simulink model "LabC_CompensatorOverRobot"  (R2020b)
settings: Solver=FixedStepDiscrete  StartTime=0.0  StopTime=inf  FixedStep=fSamplingPeriod  RelTol=1e-3  EnableMultiTasking=on
values from neighbouring files (symbols this model uses):
  acc_LSB_per_g = 16384    [GyroAccScaling.mat]
  acc_y_offset = 651.5    [OffsetData.mat]
  acc_z_offset = 170.75    [OffsetData.mat]
  Ad = Acl    [LabB_ObserverAndControllerOverSimulator_Discrete_Parameters.m]    (also in LabB_ObserverOverSimulator_Discrete_Parameters.m; LabC_6_4.m = Ad; LabC_6_5.m = Ad; LabC_6_6.m)
  Cd = [1,0,0,0 ; 0,0,1,0]    [LabB_ObserverAndControllerOverSimulator_Discrete_Parameters.m]    (also in LabB_ObserverOverSimulator_Discrete_Parameters.m; LabC_6_4.m; LabC_6_5.m; LabC_6_6.m = [1,0,0,0])
  fSamplingPeriod = 0.005    [LabB_ControllerOverSimulator_Discrete_Parameters.m]    (also in LabB_ControllerOverSimulator_Discrete_Parameters_conflict_copy_LAPTOP-FOGVCHE7_2020_11_15.m; LabB_ObserverAndControllerOverSimulator_Discrete_Parameters.m; LabC_6_3.m = 0.2; LabC_6_4.m = 0.067)
  fWheelRadius = 0.0216    [LoadRobotParameters.m]
  gyro_LSB_per_deg = 131    [GyroAccScaling.mat]
  gyro_x_offset = -193.125    [OffsetData.mat]
  iNumberOfEncoderSteps = 720    [LoadRobotParameters.m]
  Kd = place(Ad, Bd, Pd)    [LabB_ControllerOverSimulator_Discrete_Parameters.m]    (also in LabB_ControllerOverSimulator_Discrete_Parameters_conflict_copy_LAPTOP-FOGVCHE7_2020_11_15.m = c2d(K,fSamplingPeriod,'zoh'); LabB_ObserverAndControllerOverSimulator_Discrete_Parameters.m; LabC_6_6.m; LabC_CompensatorOverRobot_Parameters.m)
  Ld = (place(Ad',Cd',afPoles_full_d))'    [LabB_ObserverAndControllerOverSimulator_Discrete_Parameters.m]    (also in LabB_ObserverOverSimulator_Discrete_Parameters.m; LabC_6_4.m; LabC_6_5.m; LabC_6_6.m)
  Md1 = AXX_ - Lacc*AyX_ - Linacc*CX_    [CalcReducedObserver.m]    (also in LabB_ObserverAndControllerOverSimulator_Discrete_Parameters.m; LabB_ObserverOverSimulator_Discrete_Parameters.m; LabC_6_6.m = double(AXX_  - Linacc*CX_ ); LabC_CompensatorOverRobot_Parameters.m)
  Md2 = BX_ - Lacc*By_    [CalcReducedObserver.m]    (also in LabB_ObserverAndControllerOverSimulator_Discrete_Parameters.m; LabB_ObserverOverSimulator_Discrete_Parameters.m; LabC_6_6.m = double(BX_); LabC_CompensatorOverRobot_Parameters.m)
  Md3 = AXy_ - Lacc*Ayy_ - Linacc*Cy_    [CalcReducedObserver.m]    (also in LabB_ObserverAndControllerOverSimulator_Discrete_Parameters.m; LabB_ObserverOverSimulator_Discrete_Parameters.m; LabC_6_6.m = double(AXy_ - Linacc*Cy_); LabC_CompensatorOverRobot_Parameters.m)
  Md4 = Linacc    [CalcReducedObserver.m]    (also in LabB_ObserverAndControllerOverSimulator_Discrete_Parameters.m; LabB_ObserverOverSimulator_Discrete_Parameters.m; LabC_6_6.m = double(Linacc); LabC_CompensatorOverRobot_Parameters.m)
  Md5 = Lacc    [CalcReducedObserver.m]    (also in LabB_ObserverAndControllerOverSimulator_Discrete_Parameters.m; LabB_ObserverOverSimulator_Discrete_Parameters.m; LabC_6_6.m = double(Lacc); LabC_CompensatorOverRobot_Parameters.m)
  Md6 = T(:, 1:p)    [CalcReducedObserver.m]    (also in LabB_ObserverAndControllerOverSimulator_Discrete_Parameters.m; LabB_ObserverOverSimulator_Discrete_Parameters.m; LabC_6_6.m; LabC_CompensatorOverRobot_Parameters.m)
  Md7 = T(:, p+1:n)    [CalcReducedObserver.m]    (also in LabB_ObserverAndControllerOverSimulator_Discrete_Parameters.m; LabB_ObserverOverSimulator_Discrete_Parameters.m; LabC_6_6.m; LabC_CompensatorOverRobot_Parameters.m)
  Nud = N    [LabC_6_6.m]    (also in LabC_CompensatorOverRobot_Parameters.m = N_val; LabC_FeedbackControl_Robot_Parameters.m = 0)
  Nxd = 0    [LabC_6_6.m]    (also in LabC_CompensatorOverRobot_Parameters.m; LabC_FeedbackControl_Robot_Parameters.m)
undefined symbols (not defined in the file or in its folder): Bd, equ_offset, sigbuilder_block
libraries: MinSegLibrary_M2V3 x3, simulink x2, cstblocks x2, arduinolib x1, simulink_extras x1
settings Model: FPTRunName=FPA_Reference  SimulationMode=external  ExtModeTrigDuration=2  Creator=Alec  LastModifiedBy=janes
settings DataIOCC: SaveFormat=Array  SaveOutput=off  SignalLogging=off  DSMLogging=off  SaveTime=off  ReturnWorkspaceOutputs=off
settings OptimizationCC: PassReuseOutputArgsAs=Individual arguments  ExpressionDepthLimit=2147483647  MaxStackSize=64  EfficientTunableParamExpr=on
settings DebuggingCC: UnderspecifiedInitializationDetection=Classic  MergeDetectMultiDrivingBlocksExec=none  ParameterTunabilityLossMsg=error  StateNameClashWarn=warning  SFUnexpectedBacktrackingDiag=warning  SFNoUnconditionalDefaultTransitionDiag=warning  SFExecutionAtInitializationDiag=none  ArithmeticOperatorsInVariantConditions=warning
settings HardwareCC: ProdBitPerInt=16  ProdBitPerPointer=16  ProdBitPerSizeT=16  ProdBitPerPtrDiffT=16  ProdLargestAtomicFloat=None  ProdWordSize=8  ProdHWDeviceType=Atmel->AVR  UseEmbeddedCoderFeatures=off
settings ModelReferenceCC: PropagateSignalLabelsOutOfModel=off
settings SFSimCC: SimUseLocalCustomCode=off  MATLABDynamicMemAlloc=off  CustomCodeUndefinedFunction=UseInterfaceOnly
settings RTWCC: Description=Embedded Coder  SystemTargetFile=ert.tlc  HardwareBoard=Arduino Mega 2560  TemplateMakefile=ert_default_tmf  GenerateReport=on  RTWVerbose=off  RTWUseLocalCustomCode=off  Toolchain=Arduino AVR  BuildConfiguration=Faster Runs  IncludeHyperlinkInReport=on  LaunchReport=on  GenerateTraceInfo=on  GenerateTraceReport=on  GenerateTraceReportSl=on  GenerateTraceReportSf=on  GenerateTraceReportEml=on
settings CodeAppCC: ForceParamTrailComments=on  IgnoreCustomStorageClasses=off  OperatorAnnotations=on  SimulinkDataObjDesc=on  SFDataObjDesc=on  MATLABFcnDesc=on  CustomSymbolStrType=$N$R$M  InsertBlockDesc=on  StateflowObjectComments=on  MATLABSourceComments=on  InternalIdentifier=Classic
settings ERTTargetCC: SupportContinuousTime=on  SupportNonInlinedSFcns=on  SupportVariableSizeSignals=on
settings ConfigComp: CovMetricSettings=dw  CovSaveCumulativeToWorkspaceVar=on  CovSaveSingleToWorkspaceVar=on  CovExternalEMLEnable=off

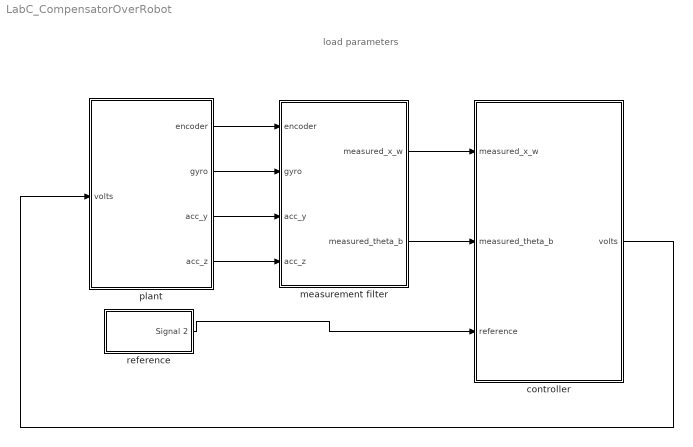
== system LabC_CompensatorOverRobot ==
  note: load parameters
  controller : Subsystem
  measurement filter : Subsystem
  plant : Subsystem
  reference : Subsystem  Tag=STV Subsys  LoadFcn=sigbuilder_block('load');  StartFcn=sigbuilder_block('start');  StopFcn=sigbuilder_block('stop');  ClipboardFcn=sigbuilder_block('clipboard');  mask(Sigbuilder block){tuvar=[0:10]}
      mask help: Simulink:masks:SigbuilderBlock_MD
      mask init:
      | if ~strcmp(get_param(bdroot(gcbh),'SimulationStatus'),'stopped') tuvar = sigbuilder_block('maskInit'); end
      settings: CopyFcn=sigbuilder_block('copy');  DeleteFcn=sigbuilder_block('delete');  ModelCloseFcn=sigbuilder_block('modelClose');  PreSaveFcn=sigbuilder_block('preSave');  PauseFcn=sigbuilder_block('pause');  ContinueFcn=sigbuilder_block('continue');  NameChangeFcn=sigbuilder_block('namechange');  OpenFcn=sigbuilder_block('open',[5.4 30 1141.2 522.6 ]);  CloseFcn=sigbuilder_block('close');
      mask Display: plot(0, 0, 100, 100,[2, 2, 32, 32, 2], [68, 8, 8, 68, 68],[32, 2], [38, 38], [32, 19, 2],[53, 60, 44], [32, 17, 17, 2],[16, 16, 31, 31]);txt = getActiveGroup(gcbh);text(2, 100, txt,'verticalAlignment', 'top');
  wires:
  controller/1(volts) -> plant/1(volts)
  measurement filter/2(measured_theta_b) -> controller/2("measured_theta_b ")
  measurement filter/1(measured_x_w) -> controller/1(measured_x_w)
  reference/1(Signal 2) -> controller/3(reference)
  plant/1(encoder) -> measurement filter/1(encoder)
  plant/2(gyro) -> measurement filter/2(gyro)
  plant/3(acc_y) -> measurement filter/3("acc_y ")
  plant/4(acc_z) -> measurement filter/4(acc_z)

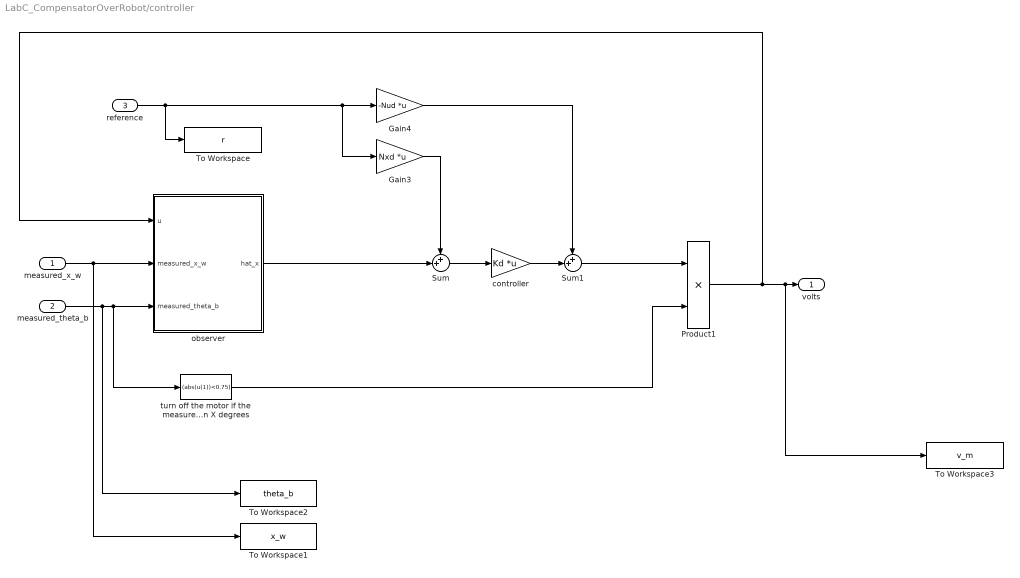
== system LabC_CompensatorOverRobot/controller ==
  measured_x_w : Inport
  "measured_theta_b " : Inport  Port=2
  reference : Inport  Port=3
  Gain3 : Gain  Gain=Nxd  Multiplication=Matrix(K*u)
  Gain4 : Gain  Gain=-Nud  Multiplication=Matrix(K*u)
  Product1 : Product  RndMeth=Zero
  Sum : Sum  Inputs=++|
  Sum1 : Sum  Inputs=++|
  To Workspace : ToWorkspace  VariableName=r  SampleTime=-1
  To Workspace1 : ToWorkspace  VariableName=x_w  SampleTime=-1
  To Workspace2 : ToWorkspace  VariableName=theta_b  SampleTime=-1
  To Workspace3 : ToWorkspace  VariableName=v_m  SampleTime=-1
  controller : Gain  Gain=Kd  Multiplication=Matrix(K*u)
  observer : Subsystem
  turn off the motor if the measured angle is greater than X degrees : Fcn  Expr=(abs(u(1))<0.75)
  volts : Outport  VectorParamsAs1DForOutWhenUnconnected=off
  wires:
  turn off the motor if the measured angle is greater than X degrees/1 -> Product1/2
  "measured_theta_b "/1 -> To Workspace2/1, observer/3(measured_theta_b), turn off the motor if the measured angle is greater than X degrees/1
  measured_x_w/1 -> observer/2(measured_x_w), To Workspace1/1
  Product1/1 -> observer/1(u), To Workspace3/1, volts/1
  Gain3/1 -> Sum/1
  Gain4/1 -> Sum1/1
  Sum/1 -> controller/1
  controller/1 -> Sum1/2
  Sum1/1 -> Product1/1
  observer/1(hat_x) -> Sum/2
  reference/1 -> To Workspace/1, Gain3/1, Gain4/1

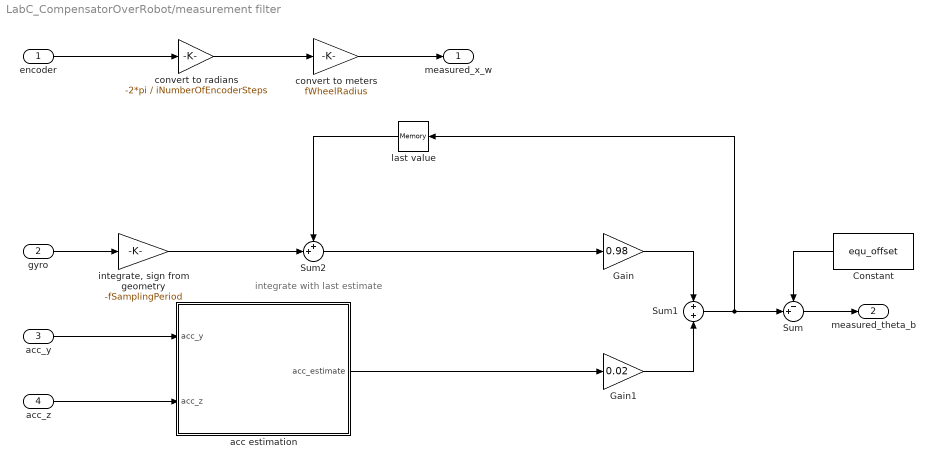
== system LabC_CompensatorOverRobot/measurement filter ==
  note: integrate with last estimate
  encoder : Inport
  gyro : Inport  Port=2
  "acc_y " : Inport  Port=3
  acc_z : Inport  Port=4
  Constant : Constant  Value=equ_offset
  Gain : Gain  Gain=0.98
  Gain1 : Gain  Gain=0.02
  Sum : Sum  Inputs=-+|
  Sum1 : Sum
  Sum2 : Sum  Inputs=++|
  acc estimation : Subsystem
  convert to radians : Gain  Gain=-2*pi / iNumberOfEncoderSteps  OutDataTypeStr=Inherit: Same as input
  convert to meters : Gain  Gain=fWheelRadius  OutDataTypeStr=Inherit: Same as input
  "integrate, sign from geometry" : Gain  Gain=-fSamplingPeriod
  last value : Memory
  measured_x_w : Outport  VectorParamsAs1DForOutWhenUnconnected=off
  measured_theta_b : Outport  Port=2  VectorParamsAs1DForOutWhenUnconnected=off
  wires:
  convert to radians/1 -> convert to meters/1
  encoder/1 -> convert to radians/1
  Sum1/1 -> Sum/2, last value/1
  convert to meters/1 -> measured_x_w/1
  "integrate, sign from geometry"/1 -> Sum2/2
  acc_z/1 -> acc estimation/2("acc_z ")
  Gain1/1 -> Sum1/2
  Sum2/1 -> Gain/1
  acc estimation/1(acc_estimate) -> Gain1/1
  Gain/1 -> Sum1/1
  gyro/1 -> "integrate, sign from geometry"/1
  last value/1 -> Sum2/1
  "acc_y "/1 -> acc estimation/1(acc_y)
  Sum/1 -> measured_theta_b/1
  Constant/1 -> Sum/1

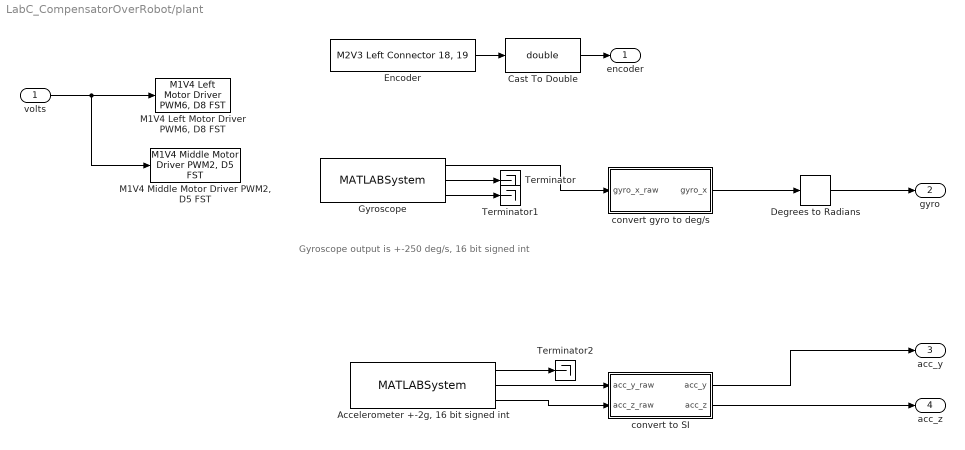
== system LabC_CompensatorOverRobot/plant ==
  note: Gyroscope output is +-250 deg/s, 16 bit signed int
  volts : Inport
  "Accelerometer +-2g, 16 bit signed int" : MATLABSystem  System=soMPU6050Accel  SimulateUsing=Code generation
      mask Type: soMPU6050Accel
      mask Display:
      | disp('soMPU6050Accel');
      | port_label('output',1,'xaccel');
      | port_label('output',2,'yaccel');
      | port_label('output',3,'zaccel');
  Cast To Double : DataTypeConversion  OutDataTypeStr=double
  Degrees to Radians : simulink_extras/Transformations/Degrees to Radians
  Encoder : MinSegLibrary_M2V3/M2V3 Left Connector 18, 19  Encoder=1  PinA=19  PinB=18
      settings: SourceProductName=Rensselaer Arduino Support Package
  Gyroscope : MATLABSystem  System=soMPU6050Gyro  DLPFmode=0
      mask Type: soMPU6050Gyro
      mask Display:
      | disp('soMPU6050Gyro');
      | port_label('output',1,'xvel');
      | port_label('output',2,'yvel');
      | port_label('output',3,'zvel');
  "M1V4 Left Motor Driver PWM6, D8 FST" : MinSegLibrary_M2V3/M1V4 Left Motor Driver PWM6, D8 FST  Vsupply=7.2
      settings: SourceProductName=Rensselaer Arduino Support Package
  "M1V4 Middle Motor Driver PWM2, D5 FST" : MinSegLibrary_M2V3/M1V4 Middle Motor Driver PWM2, D5 FST  Vsupply=7.2
      settings: SourceProductName=Rensselaer Arduino Support Package
  Terminator : Terminator
  Terminator1 : Terminator
  Terminator2 : Terminator
  convert gyro to deg/s : Subsystem
  convert to SI : Subsystem
  encoder : Outport  VectorParamsAs1DForOutWhenUnconnected=off
  gyro : Outport  Port=2  VectorParamsAs1DForOutWhenUnconnected=off
  acc_y : Outport  Port=3
  acc_z : Outport  Port=4
  wires:
  volts/1 -> "M1V4 Middle Motor Driver PWM2, D5 FST"/1, "M1V4 Left Motor Driver PWM6, D8 FST"/1
  convert to SI/1(acc_y) -> acc_y/1
  "Accelerometer +-2g, 16 bit signed int"/2 -> convert to SI/1("acc_y_raw ")
  Gyroscope/3 -> Terminator1/1
  "Accelerometer +-2g, 16 bit signed int"/1 -> Terminator2/1
  Gyroscope/1 -> convert gyro to deg/s/1(gyro_x_raw)
  "Accelerometer +-2g, 16 bit signed int"/3 -> convert to SI/2(acc_z_raw)
  convert to SI/2(acc_z) -> acc_z/1
  convert gyro to deg/s/1(gyro_x) -> Degrees to Radians/1
  Degrees to Radians/1 -> gyro/1
  Gyroscope/2 -> Terminator/1
  Encoder/1 -> Cast To Double/1
  Cast To Double/1 -> encoder/1

== system LabC_CompensatorOverRobot/reference ==
  Demux : Demux  Tag=STV Demux  Outputs=1
      settings: DisplayOption=none
  FromWs : FromWorkspace  Tag=STV FromWs  VariableName=tuvar
      SigBuilderData=|
      | common.afterFinalStr = 'Extrapolate'
      | common.sampleTime = 0
      | dataSet.timeRange = [0 120]
      | dataSet.name = 'Group 1'
      | sbobj.Groups.Name = 'Group 1'
      | sbobj.Groups.Signals.Name = 'Signal 2'
      | sbobj.Groups.Signals.XData = [0 60 60 120]
      | sbobj.Groups.Signals.YData = [0 0 1 1]
      | sbobj.Groups.TimeRange = [0 120]
  Signal 2 : Outport  Tag=STV Outport
  wires:
  FromWs/1 -> Demux/1
  Demux/1 -> Signal 2/1

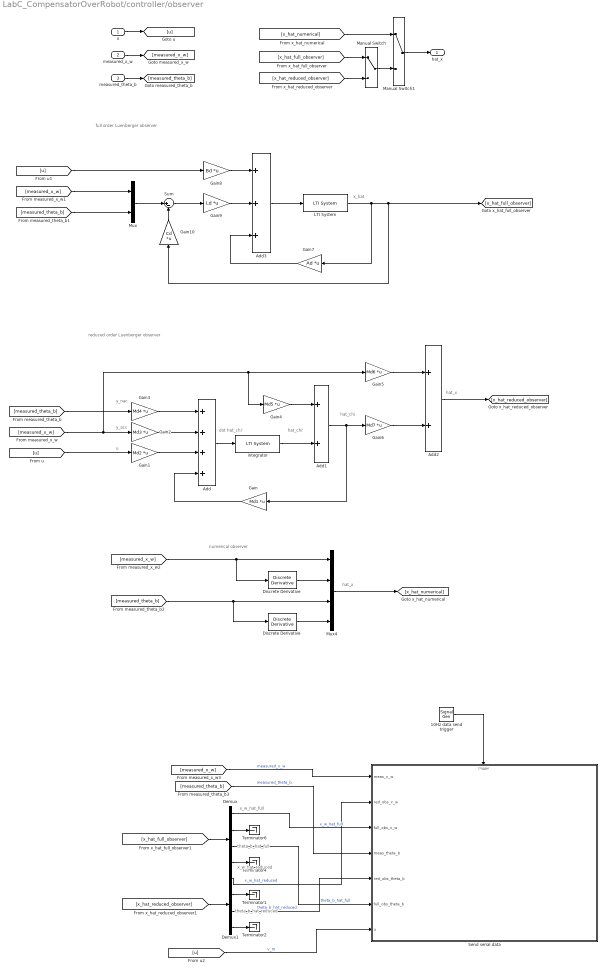
== system LabC_CompensatorOverRobot/controller/observer ==
  note: x_w_hat_full
  note: full order Luenberger observer
  note: reduced order Luenberger observer
  note: numerical observer
  note: hat_x
  note: hat_chi
  note: u
  note: dot hat_chi'
  note: hat_chi'
  note: y_acc
  note: y_nac
  note: x_hat
  note: hat_x
  note: x_w_hat_reduced
  note: theta_b_hat_full
  note: theta_b_hat_reduced
  u : Inport
  measured_x_w : Inport  Port=2
  measured_theta_b : Inport  Port=3
  10Hz data send trigger : SignalGenerator  WaveForm=sawtooth  Frequency=10
  Add : Sum  Inputs=++++
  Add1 : Sum
  Add2 : Sum
  Add3 : Sum  Inputs=+++
  Demux : Demux
  Demux1 : Demux
  Discrete Derivative : simulink/Discrete/Discrete Derivative  gainval=1.0  ICPrevScaledInput=0.0  OutMin=[]  OutMax=[]  OutDataType=fixdt(1, 16)  OutScaling=2^-10  DoSatur=off
  "Discrete Derivative " : simulink/Discrete/Discrete Derivative  gainval=1.0  ICPrevScaledInput=0.0  OutMin=[]  OutMax=[]  OutDataType=fixdt(1, 16)  OutScaling=2^-10  DoSatur=off
  Gain : Gain  Gain=Md1  Multiplication=Matrix(K*u)
  Gain1 : Gain  Gain=Md2  Multiplication=Matrix(K*u)
  Gain10 : Gain  Gain=Cd  Multiplication=Matrix(K*u)
  Gain2 : Gain  Gain=Md3  Multiplication=Matrix(K*u)
  Gain3 : Gain  Gain=Md4  Multiplication=Matrix(K*u)
  Gain4 : Gain  Gain=Md5  Multiplication=Matrix(K*u)
  Gain5 : Gain  Gain=Md6  Multiplication=Matrix(K*u)
  Gain6 : Gain  Gain=Md7  Multiplication=Matrix(K*u)
  Gain7 : Gain  Gain=Ad  Multiplication=Matrix(K*u)
  Gain8 : Gain  Gain=Bd  Multiplication=Matrix(K*u)
  Gain9 : Gain  Gain=Ld  Multiplication=Matrix(K*u)
  LTI System : cstblocks/LTI System  sys=tf(1,[1 0],fSamplingPeriod)*eye(size(Ad))  IC=[]
  Manual Switch : ManualSwitch
  Manual Switch1 : ManualSwitch
  Mux : Mux  Inputs=2
  Mux4 : Mux
  Send serial data : Subsystem  TreatAsAtomicUnit=on
  Sum : Sum  Inputs=|+-
  Terminator{1..2,4,6} (4 alike) : Terminator
  integrator : cstblocks/LTI System  sys=tf(1,[1 0],fSamplingPeriod)*eye(3)  IC=[]
  hat_x : Outport  VectorParamsAs1DForOutWhenUnconnected=off
  wires:
  Gain3/1 -> Add/1
  Gain2/1 -> Add/2
  Add/1 -> integrator/1
  Gain4/1 -> Add1/1
  Gain1/1 -> Add/3
  Gain/1 -> Add/4
  integrator/1 -> Add1/2
  Add1/1 -> Gain/1, Gain6/1
  Gain5/1 -> Add2/1
  Gain6/1 -> Add2/2
  Discrete Derivative/1 -> Mux4/2
  "Discrete Derivative "/1 -> Mux4/4
  [measured_x_w] -> Gain4/1, Gain5/1, Gain2/1
  [measured_theta_b] -> Gain3/1
  Gain9/1 -> Add3/2
  Sum/1 -> Gain9/1
  [u] -> Gain1/1
  Gain8/1 -> Add3/1
  Gain10/1 -> Sum/2
  Mux/1 -> Sum/1
  Gain7/1 -> Add3/3
  LTI System/1 -> [x_hat_full_observer], Gain10/1, Gain7/1
  Add3/1 -> LTI System/1
  u/1 -> [u]
  measured_x_w/1 -> [measured_x_w]
  measured_theta_b/1 -> [measured_theta_b]
  [u] -> Gain8/1
  [measured_x_w] -> Discrete Derivative/1, Mux4/1
  Mux4/1 -> [x_hat_numerical]
  [x_hat_full_observer] -> Manual Switch/1
  Manual Switch/1 -> Manual Switch1/2
  Manual Switch1/1 -> hat_x/1
  Add2/1 -> [x_hat_reduced_observer]
  [x_hat_reduced_observer] -> Manual Switch/2
  [x_hat_numerical] -> Manual Switch1/1
  [x_hat_full_observer] -> Demux/1
  [x_hat_reduced_observer] -> Demux1/1
  Demux/2 -> Terminator6/1
  Demux/4 -> Terminator4/1
  Demux1/2 -> Terminator1/1
  Demux1/4 -> Terminator2/1
  10Hz data send trigger/1 -> Send serial data/Trigger
  [measured_x_w] -> Send serial data/1(meas_x_w)  "measured_x_w"
  [measured_theta_b] -> Send serial data/4(meas_theta_b)  "measured_theta_b"
  Demux/1 -> Send serial data/3(full_obs_x_w)  "x_w_hat_full"
  Demux/3 -> Send serial data/6(full_obs_theta_b)  "theta_b_hat_full"
  Demux1/1 -> Send serial data/2(red_obs_x_w)  "x_w_hat_reduced"
  Demux1/3 -> Send serial data/5(red_obs_theta_b)  "theta_b_hat_reduced"
  [u] -> Send serial data/7(u)  "v_m"
  [measured_x_w] -> Mux/1
  [measured_theta_b] -> "Discrete Derivative "/1, Mux4/3
  [measured_theta_b] -> Mux/2

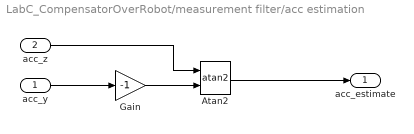
== system LabC_CompensatorOverRobot/measurement filter/acc estimation ==
  acc_y : Inport
  "acc_z " : Inport  Port=2
  Atan2 : Trigonometry  Operator=atan2
  Gain : Gain  Gain=-1
  acc_estimate : Outport  VectorParamsAs1DForOutWhenUnconnected=off
  wires:
  Gain/1 -> Atan2/2
  acc_y/1 -> Gain/1
  "acc_z "/1 -> Atan2/1
  Atan2/1 -> acc_estimate/1

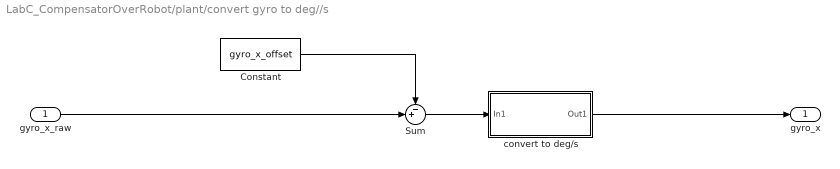
== system LabC_CompensatorOverRobot/plant/convert gyro to deg//s ==
  gyro_x_raw : Inport
  Constant : Constant  Value=gyro_x_offset
  Sum : Sum  Inputs=-+|
  convert to deg/s : Subsystem
  gyro_x : Outport  VectorParamsAs1DForOutWhenUnconnected=off
  wires:
  gyro_x_raw/1 -> Sum/2
  Sum/1 -> convert to deg/s/1(In1)
  convert to deg/s/1(Out1) -> gyro_x/1
  Constant/1 -> Sum/1

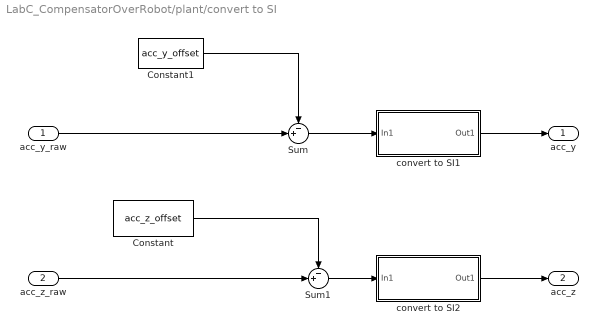
== system LabC_CompensatorOverRobot/plant/convert to SI ==
  "acc_y_raw " : Inport
  acc_z_raw : Inport  Port=2
  Constant : Constant  Value=acc_z_offset
  Constant1 : Constant  Value=acc_y_offset
  Sum : Sum  Inputs=-+|
  Sum1 : Sum  Inputs=-+|
  convert to SI1 : Subsystem
  convert to SI2 : Subsystem
  acc_y : Outport  VectorParamsAs1DForOutWhenUnconnected=off
  acc_z : Outport  Port=2  VectorParamsAs1DForOutWhenUnconnected=off
  wires:
  convert to SI1/1(Out1) -> acc_y/1
  convert to SI2/1(Out1) -> acc_z/1
  Sum/1 -> convert to SI1/1(In1)
  "acc_y_raw "/1 -> Sum/2
  Sum1/1 -> convert to SI2/1(In1)
  acc_z_raw/1 -> Sum1/2
  Constant/1 -> Sum1/1
  Constant1/1 -> Sum/1

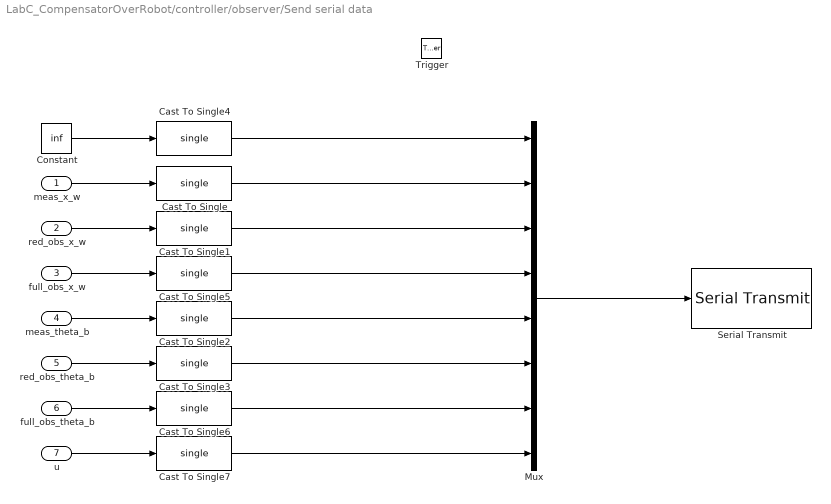
== system LabC_CompensatorOverRobot/controller/observer/Send serial data ==
  meas_x_w : Inport
  red_obs_x_w : Inport  Port=2
  full_obs_x_w : Inport  Port=3
  meas_theta_b : Inport  Port=4
  red_obs_theta_b : Inport  Port=5
  full_obs_theta_b : Inport  Port=6
  u : Inport  Port=7
  Trigger : TriggerPort  TriggerType=falling  VariantControl=Variant
  Cast To Single{,1..7} (8 alike) : DataTypeConversion  OutDataTypeStr=single
  Constant : Constant  Value=inf  OutDataTypeStr=single
  Mux : Mux  Inputs=8
  Serial Transmit : arduinolib/Serial Transmit  portNumber=0  sendmode=write  sendformat=Decimal  floatprecision=2  blockPlatform=arduino
  wires:
  Cast To Single1/1 -> Mux/3
  Cast To Single/1 -> Mux/2
  red_obs_x_w/1 -> Cast To Single1/1
  meas_x_w/1 -> Cast To Single/1
  Constant/1 -> Cast To Single4/1
  full_obs_x_w/1 -> Cast To Single5/1
  Cast To Single5/1 -> Mux/4
  Cast To Single4/1 -> Mux/1
  red_obs_theta_b/1 -> Cast To Single3/1
  full_obs_theta_b/1 -> Cast To Single6/1
  Cast To Single6/1 -> Mux/7
  meas_theta_b/1 -> Cast To Single2/1
  Cast To Single2/1 -> Mux/5
  Cast To Single3/1 -> Mux/6
  u/1 -> Cast To Single7/1
  Cast To Single7/1 -> Mux/8
  Mux/1 -> Serial Transmit/1

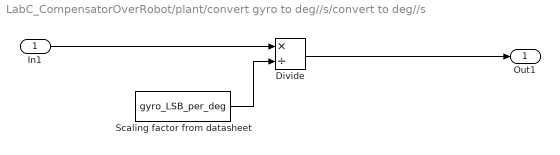
== system LabC_CompensatorOverRobot/plant/convert gyro to deg//s/convert to deg//s ==
  In1 : Inport
  Divide : Product  Inputs=*/
  Scaling factor from datasheet : Constant  Value=gyro_LSB_per_deg
  Out1 : Outport  VectorParamsAs1DForOutWhenUnconnected=off
  wires:
  Scaling factor from datasheet/1 -> Divide/2
  In1/1 -> Divide/1
  Divide/1 -> Out1/1

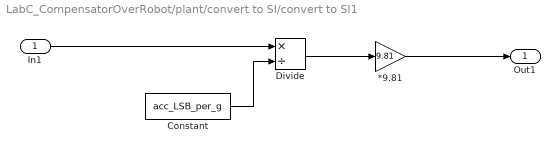
== system LabC_CompensatorOverRobot/plant/convert to SI/convert to SI1 ==
  In1 : Inport
  *9.81 : Gain  Gain=9.81
  Constant : Constant  Value=acc_LSB_per_g
  Divide : Product  Inputs=*/
  Out1 : Outport  VectorParamsAs1DForOutWhenUnconnected=off
  wires:
  Constant/1 -> Divide/2
  In1/1 -> Divide/1
  *9.81/1 -> Out1/1
  Divide/1 -> *9.81/1

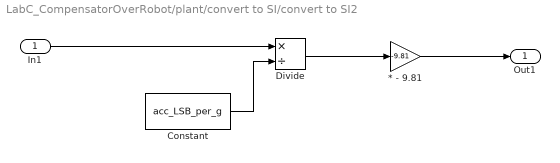
== system LabC_CompensatorOverRobot/plant/convert to SI/convert to SI2 ==
  In1 : Inport
  * - 9.81 : Gain  Gain=-9.81
  Constant : Constant  Value=acc_LSB_per_g
  Divide : Product  Inputs=*/
  Out1 : Outport  VectorParamsAs1DForOutWhenUnconnected=off
  wires:
  Constant/1 -> Divide/2
  In1/1 -> Divide/1
  * - 9.81/1 -> Out1/1
  Divide/1 -> * - 9.81/1
